simulink model "nsq_rate_lim"  (R2024b)
settings: Solver=VariableStepAuto  StartTime=0.0  StopTime=10.0  RelTol=1e-3
values from neighbouring files (symbols this model uses):
  sr = 1e4    (= 10000)    [main.m]
  Ts = 1/Fs    (= 1e-06)    [main.m]
undefined symbols (not defined in the file or in its folder): a, b
settings Model: Creator=bikashadhikari  LastModifiedBy=bikashadhikari
settings RTWCC: GPUComputeCapability=3.5

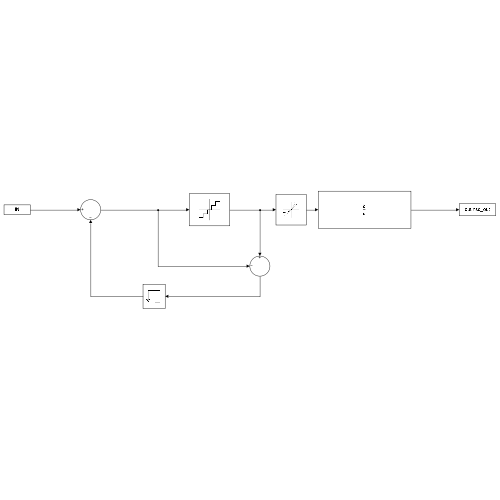
[thumbnail: Simulink's stored preview of the top-level diagram]
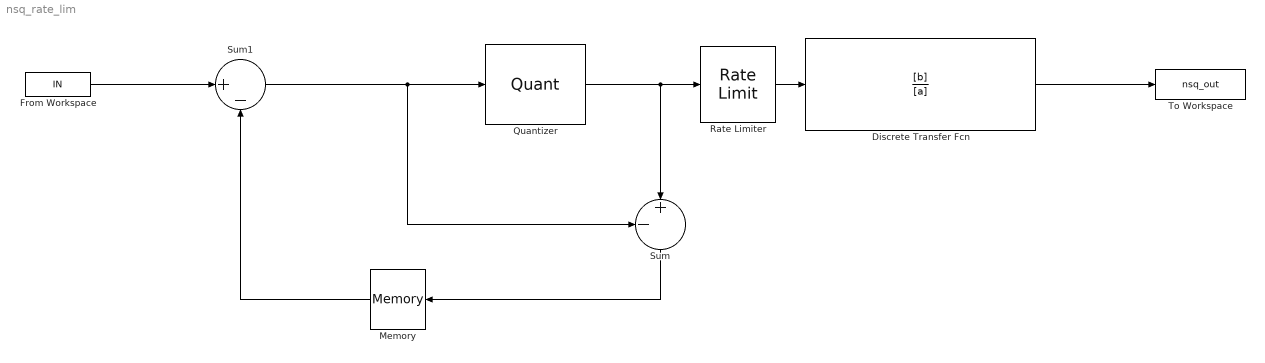
== system nsq_rate_lim ==
  Discrete Transfer Fcn : DiscreteTransferFcn  Numerator=[b]  Denominator=[a]
  From Workspace : FromWorkspace  VariableName=IN  SampleTime=Ts
  Memory : Memory
  Quantizer : Quantizer  QuantizationInterval=Qstep
  Rate Limiter : RateLimiter  RisingSlewLimit=sr  FallingSlewLimit=-sr  SampleTimeMode=inherited
  Sum : Sum  Inputs=-+|
  Sum1 : Sum  Inputs=|+-
  To Workspace : ToWorkspace  VariableName=nsq_out  SaveFormat=Timeseries  SampleTime=Ts
  wires:
  Sum/1 -> Memory/1
  Memory/1 -> Sum1/2
  From Workspace/1 -> Sum1/1
  Discrete Transfer Fcn/1 -> To Workspace/1
  Quantizer/1 -> Sum/2, Rate Limiter/1
  Rate Limiter/1 -> Discrete Transfer Fcn/1
  Sum1/1 -> Sum/1, Quantizer/1
